simulink model "loopshaping_example"  (R2018b)
settings: Solver=ode45  StartTime=0.0  StopTime=100  RelTol=1e-3  EnableMultiTasking=on
undefined symbols (not defined in the file or in its folder): ctrl, P
settings Model: Creator=beard  LastModifiedBy=beard
settings DataIOCC: LimitDataPoints=on  SaveFormat=Array
settings OptimizationCC: LifeSpan=inf
settings DebuggingCC: UnderspecifiedInitializationDetection=Classic  MergeDetectMultiDrivingBlocksExec=none  SolverPrmCheckMsg=warning  AllowSymbolicDim=off  StateNameClashWarn=warning  SFUnexpectedBacktrackingDiag=warning  SFNoUnconditionalDefaultTransitionDiag=warning  SFExecutionAtInitializationDiag=none
settings HardwareCC: ProdBitPerPointer=32  ProdBitPerSizeT=32  ProdBitPerPtrDiffT=32  ProdLargestAtomicFloat=None  ProdIntDivRoundTo=Undefined  ProdEndianess=Unspecified  ProdWordSize=32  ProdHWDeviceType=32-bit Generic
settings ModelReferenceCC: PropagateSignalLabelsOutOfModel=off
settings SFSimCC: SimUseLocalCustomCode=off
settings RTWCC: RTWUseLocalCustomCode=off
settings CodeAppCC: StateflowObjectComments=on
settings GRTTargetCC: TargetLangStandard=C89/C90 (ANSI)  GeneratePreprocessorConditionals=Disable all
settings ConfigComp: CovMetricSettings=dw  CovHtmlReporting=on  CovSaveCumulativeToWorkspaceVar=on  CovSaveSingleToWorkspaceVar=on  CovExternalEMLEnable=off

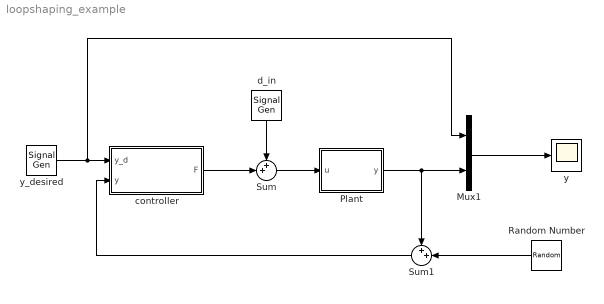
== system loopshaping_example ==
  Mux1 : Mux  Inputs=2
  Plant : Subsystem
  Random Number : RandomNumber  Variance=.01  SampleTime=P.Ts
  Sum : Sum  Inputs=++|
  Sum1 : Sum  Inputs=++|
  controller : Subsystem
  d_in : SignalGenerator  Frequency=0.1  Units=rad/sec
  y : Scope
  y_desired : SignalGenerator  WaveForm=square  Frequency=0.02
  wires:
  controller/1(F) -> Sum/2
  Plant/1(y) -> Sum1/1, Mux1/2
  Sum/1 -> Plant/1(u)
  Mux1/1 -> y/1
  y_desired/1 -> Mux1/1, controller/1(y_d)
  Sum1/1 -> controller/2(y)
  d_in/1 -> Sum/1
  Random Number/1 -> Sum1/2

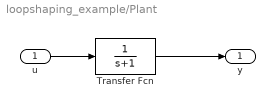
== system loopshaping_example/Plant ==
  u : Inport
  Transfer Fcn : TransferFcn  Denominator=[1 1]
  y : Outport
  wires:
  u/1 -> Transfer Fcn/1
  Transfer Fcn/1 -> y/1

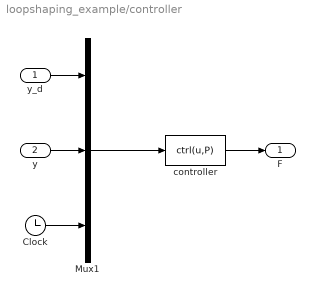
== system loopshaping_example/controller ==
  y_d : Inport
  y : Inport  Port=2
  Clock : Clock
  Mux1 : Mux  Inputs=3
  controller : MATLABFcn  MATLABFcn=ctrl(u,P)  OutputDimensions=1  SampleTime=P.Ts
  F : Outport
  wires:
  Clock/1 -> Mux1/3
  y/1 -> Mux1/2
  y_d/1 -> Mux1/1
  Mux1/1 -> controller/1
  controller/1 -> F/1
